simulink library "hal"  (Simulink 8.2)
settings: Solver=ode45  SolverMode=SingleTasking  StartTime=0.0  StopTime=10.0  RelTol=1e-3
PostLoadFcn:
  | , if any(exist('dsrtsu_mdlpostloadfcn', 'file') == [2, 3, 6]), try dsrtsu_mdlpostloadfcn('Execute', bdroot); catch fprintf('Error in PostLoadFcn (dsrtsu_mdlpostloadfcn) for model "%s":\n %s\n', bdroot, lasterr); end, end,
values from neighbouring files (symbols this model uses):
  INVALID_ABS1_TIMEOUT = single(0.03)    [hal_def.m]
  INVALID_ABS2_TIMEOUT = single(0.03)    [hal_def.m]
  INVALID_ABS3_TIMEOUT = single(0.03)    [hal_def.m]
  INVALID_ABS4_TIMEOUT = single(0.03)    [hal_def.m]
  INVALID_AC1_TIMEOUT = single(0.3)    [hal_def.m]
  INVALID_BCM1_TIMEOUT = single(0.6)    [hal_def.m]
  INVALID_BCM2_TIMEOUT = single(0.06)    [hal_def.m]
  INVALID_BOOSTER_VAC = uint32(255)    [hal_def.m]
  INVALID_CUR_VEHDECE = uint32(255)    [hal_def.m]
  INVALID_CURBRAKEDECE_REQ = uint32(255)    [hal_def.m]
  INVALID_CURSTEERANG_REQ = uint32(65535)    [hal_def.m]
  INVALID_CURSTEERTQ_REQ = uint32(255)    [hal_def.m]
  INVALID_ECM1_TIMEOUT = single(0.03)    [hal_def.m]
  INVALID_ECM2_TIMEOUT = single(0.03)    [hal_def.m]
  INVALID_ECM3_TIMEOUT = single(0.03)    [hal_def.m]
  INVALID_ECM9_TIMEOUT = single(0.03)    [hal_def.m]
  INVALID_ENG_TORQUE_FRICTIONAL = uint32(255)    [hal_def.m]
  INVALID_ENG_TORQUE_INDICATED = uint32(255)    [hal_def.m]
  INVALID_ENG_TORQUE_INDICATEDCOR = uint32(255)    [hal_def.m]
  INVALID_ENG_TQ_MAX = uint32(65535)    [hal_def.m]
  INVALID_ENG_TQ_MIN = uint32(65535)    [hal_def.m]
  INVALID_EPAS2_TIMEOUT = single(0.03)    [hal_def.m]
  INVALID_EPAS3_TIMEOUT = single(0.03)    [hal_def.m]
  INVALID_EPB1_TIMEOUT = single(0.12)    [hal_def.m]
  INVALID_EPS_BATTVOLT = uint32(251)    [hal_def.m]
  INVALID_ESC_BATTVOLT = uint32(251)    [hal_def.m]
  INVALID_GRADE = uint32(255)    [hal_def.m]
  INVALID_HCU3_TIMEOUT = single(0.03)    [hal_def.m]
  INVALID_HCU4_TIMEOUT = single(0.03)    [hal_def.m]
  INVALID_HMI1_TIMEOUT = single(0.03)    [hal_def.m]
  INVALID_HMI2_TIMEOUT = single(0.03)    [hal_def.m]
  INVALID_LAT_ACC = uint32(255)    [hal_def.m]
  INVALID_LONG_ACC = uint32(255)    [hal_def.m]
  INVALID_MC_PRESSURE = uint32(2047)    [hal_def.m]
  INVALID_METER1_TIMEOUT = single(0.3)    [hal_def.m]
  INVALID_METER3_TIMEOUT = single(0.3)    [hal_def.m]
  INVALID_METER_VEHSPD = uint32(2048)    [hal_def.m]
  INVALID_ODO_METER = uint32(1000000)    [hal_def.m]
  INVALID_OUTSIDE_TEMP = uint32(96)    [hal_def.m]
  INVALID_PARKBRAKEBIND_STAT = uint32(3)    [hal_def.m]
  INVALID_SAS1_TIMEOUT = single(0.03)    [hal_def.m]
  INVALID_SAS_ANGLE = uint32(65535)    [hal_def.m]
  INVALID_SHIFTER_POSN = uint32(6)    [hal_def.m]
  INVALID_TCM1_TIMEOUT = single(0.03)    [hal_def.m]
  INVALID_TCM2_TIMEOUT = single(0.03)    [hal_def.m]
  INVALID_VCU1_TIMEOUT = single(0.03)    [hal_def.m]
  INVALID_VCU2_TIMEOUT = single(0.03)    [hal_def.m]
  INVALID_VEH_CRASH = uint32(15)    [hal_def.m]
  INVALID_VEH_SPD = uint32(2048)    [hal_def.m]
  INVALID_WHEEL_SPD = uint32(16377)    [hal_def.m]
  INVALID_YAW_RATE = uint32(2001)    [hal_def.m]
undefined symbols (not defined in the file or in its folder): C_TASK_5MS_S, FALSE, INVALID_CURPTTORQ_REQ, KHAL_MssgIdObj1_num, KHAL_MssgIdObj2_num, KHAL_MssgIdObjStatus_num, TRUE
libraries: simulink x92
(part 5 of 8)

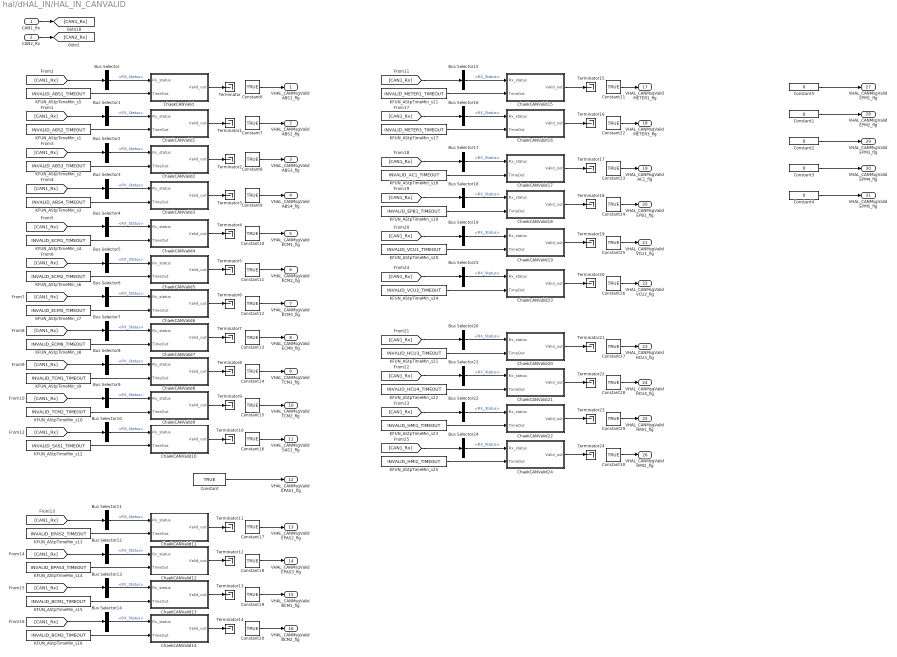
== system hal/dHAL_IN/HAL_IN_CANVALID ==
  CAN1_Rx : Inport
  CAN2_Rx : Inport  Port=2
  Bus Selector : BusSelector  OutputSignals=ABS1.RX_Status
  Bus Selector1 : BusSelector  OutputSignals=ABS2.RX_Status
  Bus Selector10 : BusSelector  OutputSignals=SAS1.RX_Status
  Bus Selector11 : BusSelector  OutputSignals=EPAS2.RX_Status
  Bus Selector12 : BusSelector  OutputSignals=EPAS3.RX_Status
  Bus Selector13 : BusSelector  OutputSignals=BCM1.RX_Status
  Bus Selector14 : BusSelector  OutputSignals=BCM2.RX_Status
  Bus Selector15 : BusSelector  OutputSignals=Meter1.RX_Status
  Bus Selector16 : BusSelector  OutputSignals=Meter3.RX_Status
  Bus Selector17 : BusSelector  OutputSignals=AC1.RX_Status
  Bus Selector18 : BusSelector  OutputSignals=EPB1.RX_Status
  Bus Selector19 : BusSelector  OutputSignals=VCU1.RX_Status
  Bus Selector2 : BusSelector  OutputSignals=ABS3.RX_Status
  Bus Selector20 : BusSelector  OutputSignals=HCU3.RX_Status
  Bus Selector21 : BusSelector  OutputSignals=HCU4.RX_Status
  Bus Selector22 : BusSelector  OutputSignals=HMI1.RX_Status
  Bus Selector23 : BusSelector  OutputSignals=VCU2.RX_Status
  Bus Selector24 : BusSelector  OutputSignals=HMI2.RX_Status
  Bus Selector3 : BusSelector  OutputSignals=ABS4.RX_Status
  Bus Selector4 : BusSelector  OutputSignals=ECM1.RX_Status
  Bus Selector5 : BusSelector  OutputSignals=ECM2.RX_Status
  Bus Selector6 : BusSelector  OutputSignals=ECM3.RX_Status
  Bus Selector7 : BusSelector  OutputSignals=ECM9.RX_Status
  Bus Selector8 : BusSelector  OutputSignals=TCM1.RX_Status
  Bus Selector9 : BusSelector  OutputSignals=TCM2.RX_Status
  ChaekCANValid : Subsystem
  ChaekCANValid1 : Subsystem
  ChaekCANValid10 : Subsystem
  ChaekCANValid11 : Subsystem
  ChaekCANValid12 : Subsystem
  ChaekCANValid13 : Subsystem
  ChaekCANValid14 : Subsystem
  ChaekCANValid15 : Subsystem
  ChaekCANValid16 : Subsystem
  ChaekCANValid17 : Subsystem
  ChaekCANValid18 : Subsystem
  ChaekCANValid19 : Subsystem
  ChaekCANValid2 : Subsystem
  ChaekCANValid20 : Subsystem
  ChaekCANValid21 : Subsystem
  ChaekCANValid22 : Subsystem
  ChaekCANValid23 : Subsystem
  ChaekCANValid24 : Subsystem
  ChaekCANValid3 : Subsystem
  ChaekCANValid4 : Subsystem
  ChaekCANValid5 : Subsystem
  ChaekCANValid6 : Subsystem
  ChaekCANValid7 : Subsystem
  ChaekCANValid8 : Subsystem
  ChaekCANValid9 : Subsystem
  Constant{,6..30} (26 alike) : Constant  Value=TRUE
  Constant{1..5} (5 alike) : Constant  Value=0
  KFUN_AStpTimeMin_s1 : Constant  Value=INVALID_ABS2_TIMEOUT
  KFUN_AStpTimeMin_s10 : Constant  Value=INVALID_TCM2_TIMEOUT
  KFUN_AStpTimeMin_s11 : Constant  Value=INVALID_METER1_TIMEOUT
  KFUN_AStpTimeMin_s12 : Constant  Value=INVALID_SAS1_TIMEOUT
  KFUN_AStpTimeMin_s13 : Constant  Value=INVALID_EPAS2_TIMEOUT
  KFUN_AStpTimeMin_s14 : Constant  Value=INVALID_EPAS3_TIMEOUT
  KFUN_AStpTimeMin_s15 : Constant  Value=INVALID_BCM1_TIMEOUT
  KFUN_AStpTimeMin_s16 : Constant  Value=INVALID_BCM2_TIMEOUT
  KFUN_AStpTimeMin_s17 : Constant  Value=INVALID_METER3_TIMEOUT
  KFUN_AStpTimeMin_s18 : Constant  Value=INVALID_AC1_TIMEOUT
  KFUN_AStpTimeMin_s19 : Constant  Value=INVALID_EPB1_TIMEOUT
  KFUN_AStpTimeMin_s2 : Constant  Value=INVALID_ABS3_TIMEOUT
  KFUN_AStpTimeMin_s20 : Constant  Value=INVALID_VCU1_TIMEOUT
  KFUN_AStpTimeMin_s21 : Constant  Value=INVALID_HCU3_TIMEOUT
  KFUN_AStpTimeMin_s22 : Constant  Value=INVALID_HCU4_TIMEOUT
  KFUN_AStpTimeMin_s23 : Constant  Value=INVALID_HMI1_TIMEOUT  VectorParams1D=off
  KFUN_AStpTimeMin_s24 : Constant  Value=INVALID_VCU2_TIMEOUT
  KFUN_AStpTimeMin_s25 : Constant  Value=INVALID_HMI2_TIMEOUT  VectorParams1D=off
  KFUN_AStpTimeMin_s3 : Constant  Value=INVALID_ABS4_TIMEOUT
  KFUN_AStpTimeMin_s4 : Constant  Value=INVALID_ECM1_TIMEOUT
  KFUN_AStpTimeMin_s5 : Constant  Value=INVALID_ABS1_TIMEOUT
  KFUN_AStpTimeMin_s6 : Constant  Value=INVALID_ECM2_TIMEOUT
  KFUN_AStpTimeMin_s7 : Constant  Value=INVALID_ECM3_TIMEOUT
  KFUN_AStpTimeMin_s8 : Constant  Value=INVALID_ECM9_TIMEOUT
  KFUN_AStpTimeMin_s9 : Constant  Value=INVALID_TCM1_TIMEOUT
  Terminator{,1..24} (25 alike) : Terminator
  VHAL_CANMsgValidABS1_flg : Outport
  VHAL_CANMsgValidABS2_flg : Outport  Port=2
  VHAL_CANMsgValidABS3_flg : Outport  Port=3
  VHAL_CANMsgValidABS4_flg : Outport  Port=4
  VHAL_CANMsgValidECM1_flg : Outport  Port=5
  VHAL_CANMsgValidECM2_flg : Outport  Port=6
  VHAL_CANMsgValidECM3_flg : Outport  Port=7
  VHAL_CANMsgValidECM9_flg : Outport  Port=8
  VHAL_CANMsgValidTCM1_flg : Outport  Port=9
  VHAL_CANMsgValidTCM2_flg : Outport  Port=10
  VHAL_CANMsgValidSAS1_flg : Outport  Port=11
  VHAL_CANMsgValidEPAS1_flg : Outport  Port=12
  VHAL_CANMsgValidEPAS2_flg : Outport  Port=13
  VHAL_CANMsgValidEPAS3_flg : Outport  Port=14
  VHAL_CANMsgValidBCM1_flg : Outport  Port=15
  VHAL_CANMsgValidBCM2_flg : Outport  Port=16
  VHAL_CANMsgValidMETER1_flg : Outport  Port=17
  VHAL_CANMsgValidMETER3_flg : Outport  Port=18
  VHAL_CANMsgValidAC1_flg : Outport  Port=19
  VHAL_CANMsgValidEPB1_flg : Outport  Port=20
  VHAL_CANMsgValidVCU1_flg : Outport  Port=21
  VHAL_CANMsgValidVCU2_flg : Outport  Port=22
  VHAL_CANMsgValidHCU3_flg : Outport  Port=23
  VHAL_CANMsgValidHCU4_flg : Outport  Port=24
  VHAL_CANMsgValidHMI1_flg : Outport  Port=25
  VHAL_CANMsgValidHMI2_flg : Outport  Port=26
  VHAL_CANMsgValidEPM1_flg : Outport  Port=27
  VHAL_CANMsgValidEPM2_flg : Outport  Port=28
  VHAL_CANMsgValidEPM3_flg : Outport  Port=29
  VHAL_CANMsgValidEPM4_flg : Outport  Port=30
  VHAL_CANMsgValidEPM5_flg : Outport  Port=31
  wires:
  Constant/1 -> VHAL_CANMsgValidEPAS1_flg/1
  Constant3/1 -> VHAL_CANMsgValidEPM4_flg/1
  Constant2/1 -> VHAL_CANMsgValidEPM3_flg/1
  Constant1/1 -> VHAL_CANMsgValidEPM2_flg/1
  Constant5/1 -> VHAL_CANMsgValidEPM1_flg/1
  Constant4/1 -> VHAL_CANMsgValidEPM5_flg/1
  [CAN1_Rx] -> Bus Selector/1
  Bus Selector/1 -> ChaekCANValid/1(Rx_status)  "<RX_Status>"
  KFUN_AStpTimeMin_s5/1 -> ChaekCANValid/2(TimeOut)
  CAN1_Rx/1 -> [CAN1_Rx]
  [CAN1_Rx] -> Bus Selector1/1
  Bus Selector1/1 -> ChaekCANValid1/1(Rx_status)  "<RX_Status>"
  KFUN_AStpTimeMin_s1/1 -> ChaekCANValid1/2(TimeOut)
  [CAN1_Rx] -> Bus Selector2/1
  Bus Selector2/1 -> ChaekCANValid2/1(Rx_status)  "<RX_Status>"
  KFUN_AStpTimeMin_s2/1 -> ChaekCANValid2/2(TimeOut)
  [CAN1_Rx] -> Bus Selector3/1
  Bus Selector3/1 -> ChaekCANValid3/1(Rx_status)  "<RX_Status>"
  KFUN_AStpTimeMin_s3/1 -> ChaekCANValid3/2(TimeOut)
  [CAN1_Rx] -> Bus Selector4/1
  Bus Selector4/1 -> ChaekCANValid4/1(Rx_status)  "<RX_Status>"
  KFUN_AStpTimeMin_s4/1 -> ChaekCANValid4/2(TimeOut)
  [CAN1_Rx] -> Bus Selector5/1
  Bus Selector5/1 -> ChaekCANValid5/1(Rx_status)  "<RX_Status>"
  KFUN_AStpTimeMin_s6/1 -> ChaekCANValid5/2(TimeOut)
  [CAN1_Rx] -> Bus Selector6/1
  Bus Selector6/1 -> ChaekCANValid6/1(Rx_status)  "<RX_Status>"
  KFUN_AStpTimeMin_s7/1 -> ChaekCANValid6/2(TimeOut)
  [CAN1_Rx] -> Bus Selector7/1
  Bus Selector7/1 -> ChaekCANValid7/1(Rx_status)  "<RX_Status>"
  KFUN_AStpTimeMin_s8/1 -> ChaekCANValid7/2(TimeOut)
  [CAN1_Rx] -> Bus Selector8/1
  Bus Selector8/1 -> ChaekCANValid8/1(Rx_status)  "<RX_Status>"
  KFUN_AStpTimeMin_s9/1 -> ChaekCANValid8/2(TimeOut)
  [CAN1_Rx] -> Bus Selector9/1
  Bus Selector9/1 -> ChaekCANValid9/1(Rx_status)  "<RX_Status>"
  KFUN_AStpTimeMin_s10/1 -> ChaekCANValid9/2(TimeOut)
  [CAN1_Rx] -> Bus Selector10/1
  Bus Selector10/1 -> ChaekCANValid10/1(Rx_status)  "<RX_Status>"
  KFUN_AStpTimeMin_s12/1 -> ChaekCANValid10/2(TimeOut)
  [CAN1_Rx] -> Bus Selector11/1
  Bus Selector11/1 -> ChaekCANValid11/1(Rx_status)  "<RX_Status>"
  KFUN_AStpTimeMin_s13/1 -> ChaekCANValid11/2(TimeOut)
  [CAN1_Rx] -> Bus Selector12/1
  Bus Selector12/1 -> ChaekCANValid12/1(Rx_status)  "<RX_Status>"
  KFUN_AStpTimeMin_s14/1 -> ChaekCANValid12/2(TimeOut)
  [CAN1_Rx] -> Bus Selector13/1
  Bus Selector13/1 -> ChaekCANValid13/1(Rx_status)  "<RX_Status>"
  KFUN_AStpTimeMin_s15/1 -> ChaekCANValid13/2(TimeOut)
  [CAN1_Rx] -> Bus Selector14/1
  Bus Selector14/1 -> ChaekCANValid14/1(Rx_status)  "<RX_Status>"
  KFUN_AStpTimeMin_s16/1 -> ChaekCANValid14/2(TimeOut)
  [CAN1_Rx] -> Bus Selector15/1
  Bus Selector15/1 -> ChaekCANValid15/1(Rx_status)  "<RX_Status>"
  KFUN_AStpTimeMin_s11/1 -> ChaekCANValid15/2(TimeOut)
  [CAN1_Rx] -> Bus Selector16/1
  Bus Selector16/1 -> ChaekCANValid16/1(Rx_status)  "<RX_Status>"
  KFUN_AStpTimeMin_s17/1 -> ChaekCANValid16/2(TimeOut)
  [CAN1_Rx] -> Bus Selector17/1
  Bus Selector17/1 -> ChaekCANValid17/1(Rx_status)  "<RX_Status>"
  KFUN_AStpTimeMin_s18/1 -> ChaekCANValid17/2(TimeOut)
  [CAN1_Rx] -> Bus Selector18/1
  Bus Selector18/1 -> ChaekCANValid18/1(Rx_status)  "<RX_Status>"
  KFUN_AStpTimeMin_s19/1 -> ChaekCANValid18/2(TimeOut)
  [CAN1_Rx] -> Bus Selector19/1
  Bus Selector19/1 -> ChaekCANValid19/1(Rx_status)  "<RX_Status>"
  KFUN_AStpTimeMin_s20/1 -> ChaekCANValid19/2(TimeOut)
  [CAN1_Rx] -> Bus Selector20/1
  Bus Selector20/1 -> ChaekCANValid20/1(Rx_status)  "<RX_Status>"
  KFUN_AStpTimeMin_s21/1 -> ChaekCANValid20/2(TimeOut)
  [CAN1_Rx] -> Bus Selector21/1
  Bus Selector21/1 -> ChaekCANValid21/1(Rx_status)  "<RX_Status>"
  KFUN_AStpTimeMin_s22/1 -> ChaekCANValid21/2(TimeOut)
  [CAN1_Rx] -> Bus Selector22/1
  Bus Selector22/1 -> ChaekCANValid22/1(Rx_status)  "<RX_Status>"
  KFUN_AStpTimeMin_s23/1 -> ChaekCANValid22/2(TimeOut)
  [CAN1_Rx] -> Bus Selector23/1
  Bus Selector23/1 -> ChaekCANValid23/1(Rx_status)  "<RX_Status>"
  KFUN_AStpTimeMin_s24/1 -> ChaekCANValid23/2(TimeOut)
  CAN2_Rx/1 -> [CAN2_Rx]
  [CAN1_Rx] -> Bus Selector24/1
  Bus Selector24/1 -> ChaekCANValid24/1(Rx_status)  "<RX_Status>"
  KFUN_AStpTimeMin_s25/1 -> ChaekCANValid24/2(TimeOut)
  ChaekCANValid/1(Valid_out) -> Terminator/1
  Constant6/1 -> VHAL_CANMsgValidABS1_flg/1
  ChaekCANValid1/1(Valid_out) -> Terminator1/1
  Constant7/1 -> VHAL_CANMsgValidABS2_flg/1
  Constant8/1 -> VHAL_CANMsgValidABS3_flg/1
  ChaekCANValid2/1(Valid_out) -> Terminator2/1
  Constant9/1 -> VHAL_CANMsgValidABS4_flg/1
  ChaekCANValid3/1(Valid_out) -> Terminator3/1
  Constant10/1 -> VHAL_CANMsgValidECM1_flg/1
  ChaekCANValid4/1(Valid_out) -> Terminator4/1
  Constant11/1 -> VHAL_CANMsgValidECM2_flg/1
  ChaekCANValid5/1(Valid_out) -> Terminator5/1
  ChaekCANValid6/1(Valid_out) -> Terminator6/1
  Constant12/1 -> VHAL_CANMsgValidECM3_flg/1
  Constant13/1 -> VHAL_CANMsgValidECM9_flg/1
  ChaekCANValid7/1(Valid_out) -> Terminator7/1
  Constant14/1 -> VHAL_CANMsgValidTCM1_flg/1
  ChaekCANValid8/1(Valid_out) -> Terminator8/1
  Constant15/1 -> VHAL_CANMsgValidTCM2_flg/1
  ChaekCANValid9/1(Valid_out) -> Terminator9/1
  Constant16/1 -> VHAL_CANMsgValidSAS1_flg/1
  ChaekCANValid10/1(Valid_out) -> Terminator10/1
  Constant17/1 -> VHAL_CANMsgValidEPAS2_flg/1
  ChaekCANValid11/1(Valid_out) -> Terminator11/1
  Constant18/1 -> VHAL_CANMsgValidEPAS3_flg/1
  ChaekCANValid12/1(Valid_out) -> Terminator12/1
  Constant19/1 -> VHAL_CANMsgValidBCM1_flg/1
  ChaekCANValid13/1(Valid_out) -> Terminator13/1
  Constant20/1 -> VHAL_CANMsgValidBCM2_flg/1
  ChaekCANValid14/1(Valid_out) -> Terminator14/1
  Constant21/1 -> VHAL_CANMsgValidMETER1_flg/1
  ChaekCANValid15/1(Valid_out) -> Terminator15/1
  Constant22/1 -> VHAL_CANMsgValidMETER3_flg/1
  ChaekCANValid16/1(Valid_out) -> Terminator16/1
  Constant23/1 -> VHAL_CANMsgValidAC1_flg/1
  ChaekCANValid17/1(Valid_out) -> Terminator17/1
  Constant24/1 -> VHAL_CANMsgValidEPB1_flg/1
  ChaekCANValid18/1(Valid_out) -> Terminator18/1
  Constant25/1 -> VHAL_CANMsgValidVCU1_flg/1
  ChaekCANValid19/1(Valid_out) -> Terminator19/1
  Constant26/1 -> VHAL_CANMsgValidVCU2_flg/1
  ChaekCANValid23/1(Valid_out) -> Terminator20/1
  Constant27/1 -> VHAL_CANMsgValidHCU3_flg/1
  ChaekCANValid20/1(Valid_out) -> Terminator21/1
  Constant28/1 -> VHAL_CANMsgValidHCU4_flg/1
  ChaekCANValid21/1(Valid_out) -> Terminator22/1
  Constant29/1 -> VHAL_CANMsgValidHMI1_flg/1
  ChaekCANValid22/1(Valid_out) -> Terminator23/1
  Constant30/1 -> VHAL_CANMsgValidHMI2_flg/1
  ChaekCANValid24/1(Valid_out) -> Terminator24/1

== system hal/dHAL_IN/HAL_IN_EPB ==
  CAN1_Rx : Inport
  BO__928_EPB1__8_EPB : Subsystem
  KFUN_AStpTimeMin_s3 : Constant  Value=INVALID_PARKBRAKEBIND_STAT
  Relational Operator3 : RelationalOperator  Operator===  OutDataTypeStr=boolean
  VHAL_ParkBrakeBindSta_enum : Outport
  VHAL_ParkBrakeBindStaInvalid_flg : Outport  Port=2
  wires:
  [CAN1_Rx] -> BO__928_EPB1__8_EPB/1(CAN1_Rx)
  CAN1_Rx/1 -> [CAN1_Rx]
  BO__928_EPB1__8_EPB/1(PB_BrakeBinStat) -> VHAL_ParkBrakeBindSta_enum/1, Relational Operator3/1
  Relational Operator3/1 -> VHAL_ParkBrakeBindStaInvalid_flg/1
  KFUN_AStpTimeMin_s3/1 -> Relational Operator3/2

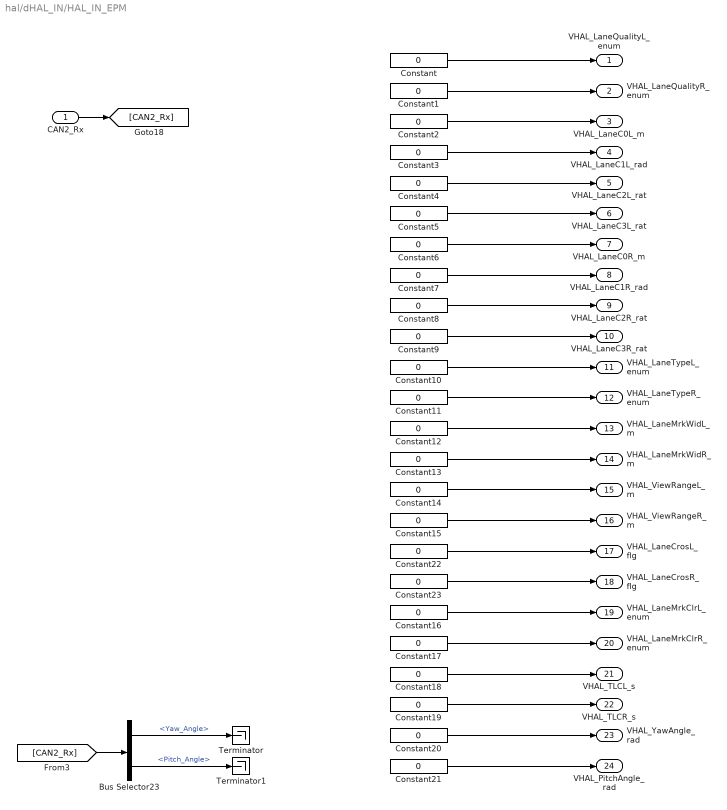
== system hal/dHAL_IN/HAL_IN_EPM ==
  CAN2_Rx : Inport
  Bus Selector23 : BusSelector  OutputSignals=Lane_Details.Yaw_Angle,Lane_Details.Pitch_Angle
  Constant{,1..23} (24 alike) : Constant  Value=0
  Terminator : Terminator
  Terminator1 : Terminator
  VHAL_LaneQualityL_enum : Outport
  VHAL_LaneQualityR_enum : Outport  Port=2
  VHAL_LaneC0L_m : Outport  Port=3
  VHAL_LaneC1L_rad : Outport  Port=4
  VHAL_LaneC2L_rat : Outport  Port=5
  VHAL_LaneC3L_rat : Outport  Port=6
  VHAL_LaneC0R_m : Outport  Port=7
  VHAL_LaneC1R_rad : Outport  Port=8
  VHAL_LaneC2R_rat : Outport  Port=9
  VHAL_LaneC3R_rat : Outport  Port=10
  VHAL_LaneTypeL_enum : Outport  Port=11
  VHAL_LaneTypeR_enum : Outport  Port=12
  VHAL_LaneMrkWidL_m : Outport  Port=13
  VHAL_LaneMrkWidR_m : Outport  Port=14
  VHAL_ViewRangeL_m : Outport  Port=15
  VHAL_ViewRangeR_m : Outport  Port=16
  VHAL_LaneCrosL_flg : Outport  Port=17
  VHAL_LaneCrosR_flg : Outport  Port=18
  VHAL_LaneMrkClrL_enum : Outport  Port=19
  VHAL_LaneMrkClrR_enum : Outport  Port=20
  VHAL_TLCL_s : Outport  Port=21
  VHAL_TLCR_s : Outport  Port=22
  VHAL_YawAngle_rad : Outport  Port=23
  VHAL_PitchAngle_rad : Outport  Port=24
  wires:
  Bus Selector23/2 -> Terminator1/1  "<Pitch_Angle>"
  Bus Selector23/1 -> Terminator/1  "<Yaw_Angle>"
  [CAN2_Rx] -> Bus Selector23/1
  CAN2_Rx/1 -> [CAN2_Rx]
  Constant21/1 -> VHAL_PitchAngle_rad/1
  Constant20/1 -> VHAL_YawAngle_rad/1
  Constant19/1 -> VHAL_TLCR_s/1
  Constant18/1 -> VHAL_TLCL_s/1
  Constant17/1 -> VHAL_LaneMrkClrR_enum/1
  Constant16/1 -> VHAL_LaneMrkClrL_enum/1
  Constant23/1 -> VHAL_LaneCrosR_flg/1
  Constant22/1 -> VHAL_LaneCrosL_flg/1
  Constant15/1 -> VHAL_ViewRangeR_m/1
  Constant14/1 -> VHAL_ViewRangeL_m/1
  Constant13/1 -> VHAL_LaneMrkWidR_m/1
  Constant12/1 -> VHAL_LaneMrkWidL_m/1
  Constant11/1 -> VHAL_LaneTypeR_enum/1
  Constant10/1 -> VHAL_LaneTypeL_enum/1
  Constant9/1 -> VHAL_LaneC3R_rat/1
  Constant8/1 -> VHAL_LaneC2R_rat/1
  Constant7/1 -> VHAL_LaneC1R_rad/1
  Constant6/1 -> VHAL_LaneC0R_m/1
  Constant5/1 -> VHAL_LaneC3L_rat/1
  Constant4/1 -> VHAL_LaneC2L_rat/1
  Constant3/1 -> VHAL_LaneC1L_rad/1
  Constant2/1 -> VHAL_LaneC0L_m/1
  Constant1/1 -> VHAL_LaneQualityR_enum/1
  Constant/1 -> VHAL_LaneQualityL_enum/1

== system hal/dHAL_IN/HAL_IN_HMI ==
  CAN1_Rx : Inport
  BO__1347_HMI1__8_HMI : Subsystem
  Detect Change{,1..2,5..8} (7 alike) : simulink/Logic and Bit Operations/Detect Change  vinit=0  InputProcessing=Inherited  OutDataTypeStr=boolean
  VHAL_AEBEnableH_flg : Outport
  VHAL_FCWEnableH_flg : Outport  Port=2
  VHAL_CSCEnableH_flg : Outport  Port=3
  VHAL_LKAEnableH_flg : Outport  Port=4
  VHAL_MAPAEnableH_flg : Outport  Port=5
  VHAL_LCSEnableH_flg : Outport  Port=6
  VHAL_LFCPilotOnH_flg : Outport  Port=7
  VHAL_LFCPilotCancelH_flg : Outport  Port=8
  VHAL_ACCOnH_flg : Outport  Port=9
  VHAL_ACCCancelH_flg : Outport  Port=10
  VHAL_ACCResSpdIncH_flg : Outport  Port=11
  VHAL_ACCSetSpdDecH_flg : Outport  Port=12
  VHAL_ACCSpdIncH_flg : Outport  Port=13
  VHAL_ACCSpdDecH_flg : Outport  Port=14
  VHAL_ACCTimeGapIncH_flg : Outport  Port=15
  VHAL_ACCTimeGapDecH_flg : Outport  Port=16
  VHAL_IGSAOnH_flg : Outport  Port=17
  VHAL_IGSAResSpdIncH_flg : Outport  Port=18
  VHAL_IGSASetSpdDecH_flg : Outport  Port=19
  VHAL_IGSASwitchModeH_flg : Outport  Port=20
  VHAL_FCWWarningModeH_enum : Outport  Port=21
  VHAL_DefMaxACCSetSpeed_kph : Outport  Port=22
  wires:
  BO__1347_HMI1__8_HMI/22(DefMaxACCSetSpeed) -> VHAL_DefMaxACCSetSpeed_kph/1
  BO__1347_HMI1__8_HMI/21(FCWWarningMode) -> VHAL_FCWWarningModeH_enum/1
  Detect Change8/1 -> VHAL_IGSASetSpdDecH_flg/1
  Detect Change7/1 -> VHAL_IGSAResSpdIncH_flg/1
  Detect Change6/1 -> VHAL_ACCTimeGapIncH_flg/1
  Detect Change5/1 -> VHAL_ACCTimeGapDecH_flg/1
  BO__1347_HMI1__8_HMI/6(ACCSpeedInc) -> VHAL_ACCSpdIncH_flg/1
  BO__1347_HMI1__8_HMI/5(ACCSpeedDec) -> VHAL_ACCSpdDecH_flg/1
  Detect Change2/1 -> VHAL_ACCSetSpdDecH_flg/1
  Detect Change1/1 -> VHAL_ACCResSpdIncH_flg/1
  Detect Change/1 -> VHAL_ACCCancelH_flg/1
  [CAN1_Rx] -> BO__1347_HMI1__8_HMI/1(CAN1_Rx)
  CAN1_Rx/1 -> [CAN1_Rx]
  BO__1347_HMI1__8_HMI/20(MAPAEnable) -> VHAL_MAPAEnableH_flg/1
  BO__1347_HMI1__8_HMI/19(LKAEnable) -> VHAL_LKAEnableH_flg/1
  BO__1347_HMI1__8_HMI/18(LFC_PilotOn) -> VHAL_LFCPilotOnH_flg/1
  BO__1347_HMI1__8_HMI/17(LFC_PilotCancel) -> VHAL_LFCPilotCancelH_flg/1
  BO__1347_HMI1__8_HMI/16(LCSEnable) -> VHAL_LCSEnableH_flg/1
  BO__1347_HMI1__8_HMI/15(IGSASwitchMode) -> VHAL_IGSASwitchModeH_flg/1
  BO__1347_HMI1__8_HMI/14(IGSASet_SpdDec) -> Detect Change8/1
  BO__1347_HMI1__8_HMI/13(IGSARes_SpdInc) -> Detect Change7/1
  BO__1347_HMI1__8_HMI/12(IGSAOn) -> VHAL_IGSAOnH_flg/1
  BO__1347_HMI1__8_HMI/11(FCWEnable) -> VHAL_FCWEnableH_flg/1
  BO__1347_HMI1__8_HMI/10(CSCEnable) -> VHAL_CSCEnableH_flg/1
  BO__1347_HMI1__8_HMI/9(AEBEnable) -> VHAL_AEBEnableH_flg/1
  BO__1347_HMI1__8_HMI/8(ACCTimeGapInc) -> Detect Change6/1
  BO__1347_HMI1__8_HMI/7(ACCTimeGapDec) -> Detect Change5/1
  BO__1347_HMI1__8_HMI/4(ACCSet_SpdDec) -> Detect Change2/1
  BO__1347_HMI1__8_HMI/3(ACCRes_SpdInc) -> Detect Change1/1
  BO__1347_HMI1__8_HMI/2(ACCOn) -> VHAL_ACCOnH_flg/1
  BO__1347_HMI1__8_HMI/1(ACCCancel) -> Detect Change/1

== system hal/dHAL_IN/HAL_IN_RadObjDecoder ==
  CAN2_Rx : Inport
  Bus Selector : BusSelector  OutputSignals=RTICANMMCaptureMessage_1.Status,RTICANMMCaptureMessage_2.Status,RTICANMMCaptureMessage_3.Status,RTICANMMCaptureMessage_4.Status,RTICANMMCaptureMessage_5.Status,RTICANMMCaptureMessage_6.Status,RTICANMMCaptureMessage_7.Status,RTICANMMCaptureMessage_8.Status,RTICANMMCaptureMessage_9.Status,RTICANMMCaptureMessage_10.Status,RTICANMMCaptureMessage_11.Status,RTICANMMCaptureMessage_12.Status,RTICANMMCaptureMessage_13.Status,RTICANMMCaptureMessage_14.Status,RTICANMMCaptureMessage_15.Status,RTICANMMCaptureMessage_16.Status,RTICANMMCaptureMessage_17.Status,RTICANMMCaptureMessage_18.Status,RTICANMMCaptureMessage_19.Status,RTICANMMCaptureMessage_20.Status,RTICANMMCaptureMessage_21.Status,RTICANMMCaptureMessage_22.Status,RTICANMMCaptureMessage_23.Status,RTICANMMCaptureMessage_24.Status,RTICANMMCaptureMessage_25.Status
  Bus Selector1 : BusSelector  OutputSignals=RTICANMMCaptureMessage_1,RTICANMMCaptureMessage_2,RTICANMMCaptureMessage_3,RTICANMMCaptureMessage_4,RTICANMMCaptureMessage_5,RTICANMMCaptureMessage_6,RTICANMMCaptureMessage_7,RTICANMMCaptureMessage_8,RTICANMMCaptureMessage_9,RTICANMMCaptureMessage_10,RTICANMMCaptureMessage_11,RTICANMMCaptureMessage_12,RTICANMMCaptureMessage_13,RTICANMMCaptureMessage_14,RTICANMMCaptureMessage_15,RTICANMMCaptureMessage_16,RTICANMMCaptureMessage_17,RTICANMMCaptureMessage_18,RTICANMMCaptureMessage_19,RTICANMMCaptureMessage_20,RTICANMMCaptureMessage_21,RTICANMMCaptureMessage_22,RTICANMMCaptureMessage_23,RTICANMMCaptureMessage_24,RTICANMMCaptureMessage_25
  Bus Selector2 : BusSelector  OutputSignals=StatusFrame,Frames1,Frames2
  Ground : Ground
  N_of_CANData : Sum  Inputs=+++++++++++++++++++++++++
  RObj_Parser : Subsystem
  RObjectPackFrame : Subsystem  TreatAsAtomicUnit=on
  VHAL_RadNofObjects_num : Outport
  VHAL_MeasCounter_num : Outport  Port=2
  VHAL_SensorRxInvalid_enum : Outport  Port=3
  VHAL_SensorSupplyVoltage_V : Outport  Port=4
  VHAL_SensorDefective_enum : Outport  Port=5
  VHAL_SensorMisaligned_enum : Outport  Port=6
  VHAL_SensorSwitchedOff_enum : Outport  Port=7
  VHAL_SensorExternalDisturbed_enum : Outport  Port=8
  VHAL_SensorOutputReduced_enum : Outport  Port=9
  VHAL_LatDistToborderLeft_m : Outport  Port=10
  VHAL_LatDistToborderRight_m : Outport  Port=11
  VHAL_RadObjRolCountVect40_num : Outport  Port=12
  VHAL_RadObjIDVect40_num : Outport  Port=13
  VHAL_RadObjXDisplVect40_m : Outport  Port=14
  VHAL_RadObjVrelXVect40_mps : Outport  Port=15
  VHAL_RadObjAccelXVect40_mps2 : Outport  Port=16
  VHAL_RadObjYDisplVect40_m : Outport  Port=17
  VHAL_RadObjDynPropVect40_enum : Outport  Port=18
  VHAL_RadObjPExistVect40_enum : Outport  Port=19
  VHAL_RadObjMeasStatVect40_enum : Outport  Port=20
  VHAL_RadObjWidthVect40_m : Outport  Port=21
  VHAL_RadObjLengthVect40_m : Outport  Port=22
  VHAL_RadObjRCSVect40_num : Outport  Port=23
  VHAL_RadObjVrelYVect40_mps : Outport  Port=24
  VHAL_RadObjProbVect40_num : Outport  Port=25
  VHAL_RadWarningLevel_enum : Outport  Port=26
  VHAL_RadWarningObjID_num : Outport  Port=27
  wires:
  RObj_Parser/27(VHAL_RadWarningObjID_num) -> VHAL_RadWarningObjID_num/1
  RObj_Parser/26(VHAL_RadWarningLevel_enum) -> VHAL_RadWarningLevel_enum/1
  RObj_Parser/25(VHAL_RadObjProbVect40_num) -> VHAL_RadObjProbVect40_num/1
  RObj_Parser/24(VHAL_RadObjVrelYVect40_mps) -> VHAL_RadObjVrelYVect40_mps/1
  RObj_Parser/23(VHAL_RadObjRCSVect40_num) -> VHAL_RadObjRCSVect40_num/1
  RObj_Parser/22(VHAL_RadObjLengthVect40_m) -> VHAL_RadObjLengthVect40_m/1
  RObj_Parser/21(VHAL_RadObjWidthVect40_m) -> VHAL_RadObjWidthVect40_m/1
  RObj_Parser/20(VHAL_RadObjMeasStatVect40_enum) -> VHAL_RadObjMeasStatVect40_enum/1
  RObj_Parser/19(VHAL_RadObjPExistVect40_enum) -> VHAL_RadObjPExistVect40_enum/1
  RObj_Parser/18(VHAL_RadObjDynPropVect40_enum) -> VHAL_RadObjDynPropVect40_enum/1
  RObj_Parser/17(VHAL_RadObjYDisplVect40_m) -> VHAL_RadObjYDisplVect40_m/1
  RObj_Parser/16(VHAL_RadObjAccelXVect40_mps2) -> VHAL_RadObjAccelXVect40_mps2/1
  RObj_Parser/15(VHAL_RadObjVrelXVect40_mps) -> VHAL_RadObjVrelXVect40_mps/1
  RObj_Parser/14(VHAL_RadObjXDisplVect40_m) -> VHAL_RadObjXDisplVect40_m/1
  RObj_Parser/13(VHAL_RadObjIDVect40_num) -> VHAL_RadObjIDVect40_num/1
  RObj_Parser/12(VHAL_RadObjRolCountVect40_num) -> VHAL_RadObjRolCountVect40_num/1
  RObj_Parser/11(VHAL_LatDistToborderRight_m) -> VHAL_LatDistToborderRight_m/1
  RObj_Parser/9(VHAL_SensorOutputReduced_enum) -> VHAL_SensorOutputReduced_enum/1
  RObj_Parser/8(VHAL_SensorExternalDisturbed_enum) -> VHAL_SensorExternalDisturbed_enum/1
  RObj_Parser/2(VHAL_MeasCounter_num) -> VHAL_MeasCounter_num/1
  RObj_Parser/10(VHAL_LatDistToborderLeft_m) -> VHAL_LatDistToborderLeft_m/1
  RObj_Parser/6(VHAL_SensorMisaligned_enum) -> VHAL_SensorMisaligned_enum/1
  RObj_Parser/4(VHAL_SensorSupplyVoltage_V) -> VHAL_SensorSupplyVoltage_V/1
  RObj_Parser/7(VHAL_SensorSwitchedOff_enum) -> VHAL_SensorSwitchedOff_enum/1
  RObj_Parser/3(VHAL_SensorRxInvalid_enum) -> VHAL_SensorRxInvalid_enum/1
  RObj_Parser/1(VHAL_RadNofObjects_num) -> VHAL_RadNofObjects_num/1
  RObj_Parser/5(VHAL_SensorDefective_enum) -> VHAL_SensorDefective_enum/1
  [RObj_Frames2] -> RObj_Parser/3(RObj_Frames2)
  [RObj_Frames1] -> RObj_Parser/2(RObj_Frames1)
  [RObj_Status] -> RObj_Parser/1(RObj_Status)
  CAN2_Rx/1 -> Bus Selector/1, Bus Selector1/1
  Bus Selector2/3 -> [RObj_Frames2]  "<Frames2>"
  Bus Selector2/2 -> [RObj_Frames1]  "<Frames1>"
  Bus Selector2/1 -> [RObj_Status]  "<StatusFrame>"
  RObjectPackFrame/1(R_Objects_out) -> Bus Selector2/1
  Bus Selector1/2 -> RObjectPackFrame/3(CaptureMessage2)  "<RTICANMMCaptureMessage_2>"
  Bus Selector1/1 -> RObjectPackFrame/2(CaptureMessage1)  "<RTICANMMCaptureMessage_1>"
  Bus Selector1/8 -> RObjectPackFrame/9(CaptureMessage8)  "<RTICANMMCaptureMessage_8>"
  Bus Selector1/10 -> RObjectPackFrame/11(CaptureMessage10)  "<RTICANMMCaptureMessage_10>"
  Bus Selector1/11 -> RObjectPackFrame/12(CaptureMessage11)  "<RTICANMMCaptureMessage_11>"
  Bus Selector1/12 -> RObjectPackFrame/13(CaptureMessage12)  "<RTICANMMCaptureMessage_12>"
  Bus Selector1/9 -> RObjectPackFrame/10(CaptureMessage9)  "<RTICANMMCaptureMessage_9>"
  Bus Selector1/13 -> RObjectPackFrame/14(CaptureMessage13)  "<RTICANMMCaptureMessage_13>"
  Bus Selector1/22 -> RObjectPackFrame/23(CaptureMessage22)  "<RTICANMMCaptureMessage_22>"
  Bus Selector1/18 -> RObjectPackFrame/19(CaptureMessage18)  "<RTICANMMCaptureMessage_18>"
  Bus Selector1/17 -> RObjectPackFrame/18(CaptureMessage17)  "<RTICANMMCaptureMessage_17>"
  Bus Selector1/23 -> RObjectPackFrame/24(CaptureMessage23)  "<RTICANMMCaptureMessage_23>"
  Bus Selector1/24 -> RObjectPackFrame/25(CaptureMessage24)  "<RTICANMMCaptureMessage_24>"
  Bus Selector1/21 -> RObjectPackFrame/22(CaptureMessage21)  "<RTICANMMCaptureMessage_21>"
  Bus Selector1/19 -> RObjectPackFrame/20(CaptureMessage19)  "<RTICANMMCaptureMessage_19>"
  Bus Selector1/20 -> RObjectPackFrame/21(CaptureMessage20)  "<RTICANMMCaptureMessage_20>"
  Bus Selector1/16 -> RObjectPackFrame/17(CaptureMessage16)  "<RTICANMMCaptureMessage_16>"
  Bus Selector1/14 -> RObjectPackFrame/15(CaptureMessage14)  "<RTICANMMCaptureMessage_14>"
  Bus Selector1/15 -> RObjectPackFrame/16(CaptureMessage15)  "<RTICANMMCaptureMessage_15>"
  Bus Selector1/25 -> RObjectPackFrame/26(CaptureMessage25)  "<RTICANMMCaptureMessage_25>"
  Bus Selector1/5 -> RObjectPackFrame/6(CaptureMessage5)  "<RTICANMMCaptureMessage_5>"
  Bus Selector1/3 -> RObjectPackFrame/4(CaptureMessage3)  "<RTICANMMCaptureMessage_3>"
  Bus Selector1/6 -> RObjectPackFrame/7(CaptureMessage6)  "<RTICANMMCaptureMessage_6>"
  Bus Selector1/7 -> RObjectPackFrame/8(CaptureMessage7)  "<RTICANMMCaptureMessage_7>"
  Bus Selector1/4 -> RObjectPackFrame/5(CaptureMessage4)  "<RTICANMMCaptureMessage_4>"
  N_of_CANData/1 -> RObjectPackFrame/1(CAN_Frames)
  Bus Selector/25 -> N_of_CANData/25  "<Status>"
  Bus Selector/24 -> N_of_CANData/24  "<Status>"
  Bus Selector/23 -> N_of_CANData/23  "<Status>"
  Bus Selector/22 -> N_of_CANData/22  "<Status>"
  Bus Selector/21 -> N_of_CANData/21  "<Status>"
  Bus Selector/20 -> N_of_CANData/20  "<Status>"
  Bus Selector/19 -> N_of_CANData/19  "<Status>"
  Bus Selector/18 -> N_of_CANData/18  "<Status>"
  Bus Selector/17 -> N_of_CANData/17  "<Status>"
  Bus Selector/16 -> N_of_CANData/16  "<Status>"
  Bus Selector/15 -> N_of_CANData/15  "<Status>"
  Bus Selector/14 -> N_of_CANData/14  "<Status>"
  Bus Selector/13 -> N_of_CANData/13  "<Status>"
  Bus Selector/12 -> N_of_CANData/12  "<Status>"
  Bus Selector/11 -> N_of_CANData/11  "<Status>"
  Bus Selector/10 -> N_of_CANData/10  "<Status>"
  Bus Selector/9 -> N_of_CANData/9  "<Status>"
  Bus Selector/8 -> N_of_CANData/8  "<Status>"
  Bus Selector/7 -> N_of_CANData/7  "<Status>"
  Bus Selector/6 -> N_of_CANData/6  "<Status>"
  Bus Selector/5 -> N_of_CANData/5  "<Status>"
  Bus Selector/4 -> N_of_CANData/4  "<Status>"
  Bus Selector/3 -> N_of_CANData/3  "<Status>"
  Bus Selector/2 -> N_of_CANData/2  "<Status>"
  Bus Selector/1 -> N_of_CANData/1  "<Status>"
  Ground/1 -> RObj_Parser/4(RObj_CollDetWarn)

== system hal/dHAL_IN/HAL_IN_SBG ==
  CAN2_Rx : Inport
  Bus Selector23 : BusSelector  OutputSignals=SBG1.SBG_LONGITUDE,SBG1.SBG_LATITUDE,SBG2.SBG_UNDULATION,SBG2.SBG_ALTITUDE,SBG3.SBG_COURSE_ACC,SBG3.SBG_COURSE
  VHAL_LONGIDUTE_deg : Outport
  VHAL_LATITUDE_deg : Outport  Port=2
  VHAL_UNDULATION_m : Outport  Port=3
  VHAL_ALTITUDE_m : Outport  Port=4
  VHAL_COURSEACC_deg : Outport  Port=5
  VHAL_COURSE_deg : Outport  Port=6
  wires:
  CAN2_Rx/1 -> [CAN2_Rx]
  [CAN2_Rx] -> Bus Selector23/1
  Bus Selector23/1 -> VHAL_LONGIDUTE_deg/1  "<SBG_LONGITUDE>"
  Bus Selector23/2 -> VHAL_LATITUDE_deg/1  "<SBG_LATITUDE>"
  Bus Selector23/3 -> VHAL_UNDULATION_m/1  "<SBG_UNDULATION>"
  Bus Selector23/4 -> VHAL_ALTITUDE_m/1  "<SBG_ALTITUDE>"
  Bus Selector23/5 -> VHAL_COURSEACC_deg/1  "<SBG_COURSE_ACC>"
  Bus Selector23/6 -> VHAL_COURSE_deg/1  "<SBG_COURSE>"

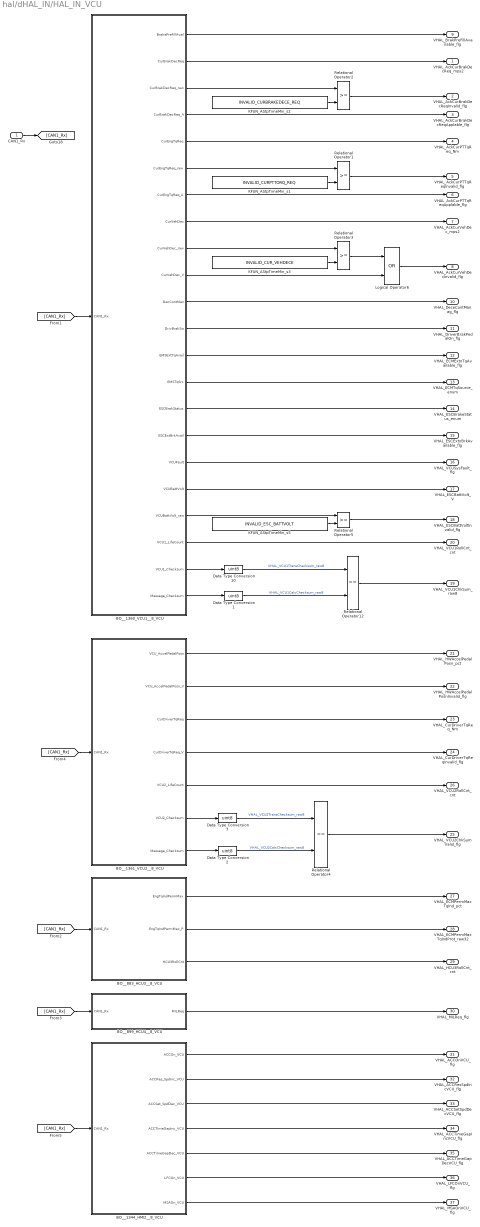
== system hal/dHAL_IN/HAL_IN_VCU ==
  CAN1_Rx : Inport
  BO__1344_HMI2__8_VCU : Subsystem
  BO__1360_VCU1__8_VCU : Subsystem
  BO__1361_VCU2__8_VCU : Subsystem
  BO__883_HCU3__8_VCU : Subsystem
  BO__899_HCU4__8_VCU : Subsystem
  Data Type Conversion{1..3,10} (4 alike) : DataTypeConversion  OutDataTypeStr=uint8
  KFUN_AStpTimeMin_s1 : Constant  Value=INVALID_CURPTTORQ_REQ
  KFUN_AStpTimeMin_s2 : Constant  Value=INVALID_CURBRAKEDECE_REQ
  KFUN_AStpTimeMin_s3 : Constant  Value=INVALID_CUR_VEHDECE
  KFUN_AStpTimeMin_s5 : Constant  Value=INVALID_ESC_BATTVOLT
  Logical Operator6 : Logic  Operator=OR  AllPortsSameDT=off  OutDataTypeStr=boolean
  Relational Operator{1..3,5} (4 alike) : RelationalOperator  OutDataTypeStr=boolean
  Relational Operator12 : RelationalOperator  Operator===  OutDataTypeStr=boolean
  Relational Operator4 : RelationalOperator  Operator===  OutDataTypeStr=boolean
  VHAL_AckCurBrakDecReq_mps2 : Outport
  VHAL_AckCurBrakDecReqInvalid_flg : Outport  Port=2
  VHAL_AckCurBrakDecReqApplable_flg : Outport  Port=3
  VHAL_AckCurPTTqReq_Nm : Outport  Port=4
  VHAL_AckCurPTTqReqInvalid_flg : Outport  Port=5
  VHAL_AckCurPTTqReqApplable_flg : Outport  Port=6
  VHAL_AckCurVehDec_mps2 : Outport  Port=7
  VHAL_AckCurVehDecInvalid_flg : Outport  Port=8
  VHAL_BrakPreFillAvailable_flg : Outport  Port=9
  VHAL_DeceContManag_flg : Outport  Port=10
  VHAL_DriverBrakPedalOn_flg : Outport  Port=11
  VHAL_ECMExtnTqAvailable_flg : Outport  Port=12
  VHAL_ECMTqSource_enum : Outport  Port=13
  VHAL_ESCBrakeStatus_enum : Outport  Port=14
  VHAL_ESCExtnBrkAvailable_flg : Outport  Port=15
  VHAL_VCUSysFault_flg : Outport  Port=16
  VHAL_ESCBattVolt_V : Outport  Port=17
  VHAL_ESCBattVoltInvalid_flg : Outport  Port=18
  VHAL_VCU1ChkSum_raw8 : Outport  Port=19
  VHAL_VCU1RollCnt_cnt : Outport  Port=20
  VHAL_HWAccelPedalPosn_pct : Outport  Port=21
  VHAL_HWAccelPedalPosnInvalid_flg : Outport  Port=22
  VHAL_CurDriverTqReq_Nm : Outport  Port=23
  VHAL_CurDriverTqReqInvalid_flg : Outport  Port=24
  VHAL_VCU2ChkSumValid_flg : Outport  Port=25
  VHAL_VCU2RollCnt_cnt : Outport  Port=26
  VHAL_ECMPermMaxTqInd_pct : Outport  Port=27
  VHAL_ECMPermMaxTqIndProt_raw32 : Outport  Port=28
  VHAL_HCU3RollCnt_cnt : Outport  Port=29
  VHAL_MILReq_flg : Outport  Port=30
  VHAL_ACCOnVCU_flg : Outport  Port=31
  VHAL_ACCResSpdIncVCU_flg : Outport  Port=32
  VHAL_ACCSetSpdDecVCU_flg : Outport  Port=33
  VHAL_ACCTimeGapIncVCU_flg : Outport  Port=34
  VHAL_ACCTimeGapDecVCU_flg : Outport  Port=35
  VHAL_LFCOnVCU_flg : Outport  Port=36
  VHAL_MSAOnVCU_flg : Outport  Port=37
  wires:
  BO__1344_HMI2__8_VCU/7(MSAOn_VCU) -> VHAL_MSAOnVCU_flg/1
  BO__1361_VCU2__8_VCU/4(CurDriverTqReq_V) -> VHAL_CurDriverTqReqInvalid_flg/1
  BO__1361_VCU2__8_VCU/3(CurDriverTqReq) -> VHAL_CurDriverTqReq_Nm/1
  BO__1361_VCU2__8_VCU/5(VCU2_LifeCount) -> VHAL_VCU2RollCnt_cnt/1
  BO__1361_VCU2__8_VCU/2(VCU_AccelPedalPosn_V) -> VHAL_HWAccelPedalPosnInvalid_flg/1
  BO__1361_VCU2__8_VCU/1(VCU_AccelPedalPosn) -> VHAL_HWAccelPedalPosn_pct/1
  BO__1361_VCU2__8_VCU/7(Message_Checksum) -> Data Type Conversion2/1
  BO__1361_VCU2__8_VCU/6(VCU2_Checksum) -> Data Type Conversion3/1
  Data Type Conversion2/1 -> Relational Operator4/2  "VHAL_VCU2CalcChecksum_raw8"
  Data Type Conversion3/1 -> Relational Operator4/1  "VHAL_VCU2TransChecksum_raw8"
  Relational Operator4/1 -> VHAL_VCU2ChkSumValid_flg/1
  [CAN1_Rx] -> BO__1361_VCU2__8_VCU/1(CAN1_Rx)
  BO__1360_VCU1__8_VCU/22(Message_Checksum) -> Data Type Conversion1/1
  BO__1360_VCU1__8_VCU/21(VCU1_Checksum) -> Data Type Conversion10/1
  Data Type Conversion1/1 -> Relational Operator12/2  "VHAL_VCU1CalcChecksum_raw8"
  Data Type Conversion10/1 -> Relational Operator12/1  "VHAL_VCU1TransChecksum_raw8"
  [CAN1_Rx] -> BO__899_HCU4__8_VCU/1(CAN1_Rx)
  [CAN1_Rx] -> BO__883_HCU3__8_VCU/1(CAN1_Rx)
  BO__1360_VCU1__8_VCU/3(CurBrakDecReq_raw) -> Relational Operator2/1
  BO__1360_VCU1__8_VCU/6(CurEngTqReq_raw) -> Relational Operator1/1
  BO__1360_VCU1__8_VCU/9(CurVehDec_raw) -> Relational Operator3/1
  BO__1360_VCU1__8_VCU/19(VCUBattVolt_raw) -> Relational Operator5/1
  [CAN1_Rx] -> BO__1360_VCU1__8_VCU/1(CAN1_Rx)
  CAN1_Rx/1 -> [CAN1_Rx]
  BO__899_HCU4__8_VCU/1(MILReq) -> VHAL_MILReq_flg/1
  BO__883_HCU3__8_VCU/3(HCU3RollCnt) -> VHAL_HCU3RollCnt_cnt/1
  BO__883_HCU3__8_VCU/2(EngTqIndPermMax_P) -> VHAL_ECMPermMaxTqIndProt_raw32/1
  BO__883_HCU3__8_VCU/1(EngTqIndPermMax) -> VHAL_ECMPermMaxTqInd_pct/1
  BO__1360_VCU1__8_VCU/20(VCU1_LifeCount) -> VHAL_VCU1RollCnt_cnt/1
  Relational Operator12/1 -> VHAL_VCU1ChkSum_raw8/1
  KFUN_AStpTimeMin_s5/1 -> Relational Operator5/2
  Relational Operator5/1 -> VHAL_ESCBattVoltInvalid_flg/1
  BO__1360_VCU1__8_VCU/18(VCUBattVolt) -> VHAL_ESCBattVolt_V/1
  BO__1360_VCU1__8_VCU/17(VCUFault) -> VHAL_VCUSysFault_flg/1
  BO__1360_VCU1__8_VCU/16(ESCExtBrkAvail) -> VHAL_ESCExtnBrkAvailable_flg/1
  BO__1360_VCU1__8_VCU/15(ESCBrakStatus) -> VHAL_ESCBrakeStatus_enum/1
  BO__1360_VCU1__8_VCU/14(EMSTqSrc) -> VHAL_ECMTqSource_enum/1
  BO__1360_VCU1__8_VCU/13(EMSExtTqAvail) -> VHAL_ECMExtnTqAvailable_flg/1
  BO__1360_VCU1__8_VCU/12(DrivBrakSw) -> VHAL_DriverBrakPedalOn_flg/1
  BO__1360_VCU1__8_VCU/11(DecContMan) -> VHAL_DeceContManag_flg/1
  BO__1360_VCU1__8_VCU/8(CurVehDec) -> VHAL_AckCurVehDec_mps2/1
  BO__1360_VCU1__8_VCU/5(CurEngTqReq) -> VHAL_AckCurPTTqReq_Nm/1
  BO__1360_VCU1__8_VCU/2(CurBrakDecReq) -> VHAL_AckCurBrakDecReq_mps2/1
  BO__1360_VCU1__8_VCU/10(CurVehDec_V) -> Logical Operator6/2
  KFUN_AStpTimeMin_s3/1 -> Relational Operator3/2
  Relational Operator3/1 -> Logical Operator6/1
  Logical Operator6/1 -> VHAL_AckCurVehDecInvalid_flg/1
  BO__1360_VCU1__8_VCU/7(CurEngTqReq_A) -> VHAL_AckCurPTTqReqApplable_flg/1
  KFUN_AStpTimeMin_s1/1 -> Relational Operator1/2
  Relational Operator1/1 -> VHAL_AckCurPTTqReqInvalid_flg/1
  BO__1360_VCU1__8_VCU/4(CurBrakDecReq_A) -> VHAL_AckCurBrakDecReqApplable_flg/1
  KFUN_AStpTimeMin_s2/1 -> Relational Operator2/2
  Relational Operator2/1 -> VHAL_AckCurBrakDecReqInvalid_flg/1
  BO__1360_VCU1__8_VCU/1(BrakePrefillAvail) -> VHAL_BrakPreFillAvailable_flg/1
  BO__1344_HMI2__8_VCU/1(ACCOn_VCU) -> VHAL_ACCOnVCU_flg/1
  BO__1344_HMI2__8_VCU/2(ACCRes_SpdInc_VCU) -> VHAL_ACCResSpdIncVCU_flg/1
  BO__1344_HMI2__8_VCU/3(ACCSet_SpdDec_VCU) -> VHAL_ACCSetSpdDecVCU_flg/1
  BO__1344_HMI2__8_VCU/5(ACCTimeGapDec_VCU) -> VHAL_ACCTimeGapDecVCU_flg/1
  BO__1344_HMI2__8_VCU/4(ACCTimeGapInc_VCU) -> VHAL_ACCTimeGapIncVCU_flg/1
  BO__1344_HMI2__8_VCU/6(LFCOn_VCU) -> VHAL_LFCOnVCU_flg/1
  [CAN1_Rx] -> BO__1344_HMI2__8_VCU/1(CAN1_Rx)

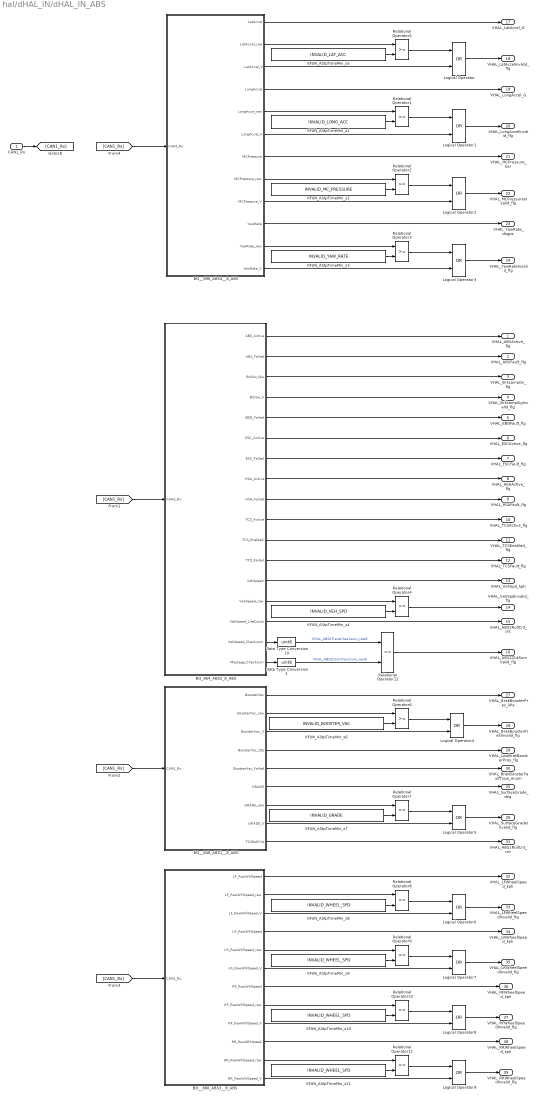
== system hal/dHAL_IN/dHAL_IN_ABS ==
  CAN1_Rx : Inport
  BO_864_ABS2_8_ABS : Subsystem
  BO__848_ABS1__8_ABS : Subsystem
  BO__880_ABS3__8_ABS : Subsystem
  BO__896_ABS4__8_ABS : Subsystem
  Data Type Conversion1 : DataTypeConversion  OutDataTypeStr=uint8
  Data Type Conversion10 : DataTypeConversion  OutDataTypeStr=uint8
  KFUN_AStpTimeMin_s1 : Constant  Value=INVALID_LONG_ACC
  KFUN_AStpTimeMin_s{8..11} (4 alike) : Constant  Value=INVALID_WHEEL_SPD
  KFUN_AStpTimeMin_s2 : Constant  Value=INVALID_MC_PRESSURE
  KFUN_AStpTimeMin_s3 : Constant  Value=INVALID_YAW_RATE
  KFUN_AStpTimeMin_s4 : Constant  Value=INVALID_VEH_SPD
  KFUN_AStpTimeMin_s5 : Constant  Value=INVALID_LAT_ACC
  KFUN_AStpTimeMin_s6 : Constant  Value=INVALID_BOOSTER_VAC
  KFUN_AStpTimeMin_s7 : Constant  Value=INVALID_GRADE
  Logical Operator{,1..9} (10 alike) : Logic  Operator=OR  AllPortsSameDT=off  OutDataTypeStr=boolean
  Relational Operator{1..11} (11 alike) : RelationalOperator  OutDataTypeStr=boolean
  Relational Operator12 : RelationalOperator  Operator===  OutDataTypeStr=boolean
  VHAL_ABSActive_flg : Outport
  VHAL_ABSFault_flg : Outport  Port=2
  VHAL_BrkLampOn_flg : Outport  Port=3
  VHAL_BrkLampSigInvalid_flg : Outport  Port=4
  VHAL_EBDFault_flg : Outport  Port=5
  VHAL_ESCActive_flg : Outport  Port=6
  VHAL_ESCFault_flg : Outport  Port=7
  VHAL_HSAActive_flg : Outport  Port=8
  VHAL_HSAFault_flg : Outport  Port=9
  VHAL_TCSActive_flg : Outport  Port=10
  VHAL_TCSEnabled_flg : Outport  Port=11
  VHAL_TCSFault_flg : Outport  Port=12
  VHAL_VehSpd_kph : Outport  Port=13
  VHAL_VehSpdInvalid_flg : Outport  Port=14
  VHAL_ABS2RollCnt_cnt : Outport  Port=15
  VHAL_ABS2ChkSumValid_flg : Outport  Port=16
  VHAL_LatAccel_G : Outport  Port=17
  VHAL_LatAccelInvalid_flg : Outport  Port=18
  VHAL_LongAccel_G : Outport  Port=19
  VHAL_LongAccelInvalid_flg : Outport  Port=20
  VHAL_MCPressure_bar : Outport  Port=21
  VHAL_MCPressureInvalid_flg : Outport  Port=22
  VHAL_YawRate_degps : Outport  Port=23
  VHAL_YawRateInvalid_flg : Outport  Port=24
  VHAL_SurfaceGrade_deg : Outport  Port=25
  VHAL_SurfaceGradeInvalid_flg : Outport  Port=26
  VHAL_BrakBoosterPres_kPa : Outport  Port=27
  VHAL_BrakBoosterPresInvalid_flg : Outport  Port=28
  VHAL_LowBrakBoosterPres_flg : Outport  Port=29
  VHAL_BrakBoosterFaultType_enum : Outport  Port=30
  VHAL_ABS1RollCnt_cnt : Outport  Port=31
  VHAL_LFWheelSpeed_kph : Outport  Port=32
  VHAL_LFWheelSpeedInvalid_flg : Outport  Port=33
  VHAL_LRWheelSpeed_kph : Outport  Port=34
  VHAL_LRWheelSpeedInvalid_flg : Outport  Port=35
  VHAL_RFWheelSpeed_kph : Outport  Port=36
  VHAL_RFWheelSpeedInvalid_flg : Outport  Port=37
  VHAL_RRWheelSpeed_kph : Outport  Port=38
  VHAL_RRWheelSpeedInvalid_flg : Outport  Port=39
  wires:
  BO__880_ABS3__8_ABS/2(LF_RawWhlSpeed_raw) -> Relational Operator8/1
  BO__880_ABS3__8_ABS/5(LR_RawWhlSpeed_raw) -> Relational Operator9/1
  BO__880_ABS3__8_ABS/8(RF_RawWhlSpeed_raw) -> Relational Operator10/1
  BO__880_ABS3__8_ABS/11(RR_RawWhlSpeed_raw) -> Relational Operator11/1
  BO__848_ABS1__8_ABS/7(GRADE_raw) -> Relational Operator7/1
  Relational Operator6/1 -> Logical Operator4/1
  BO__848_ABS1__8_ABS/2(BoosterVac_raw) -> Relational Operator6/1
  BO_864_ABS2_8_ABS/14(VehSpeed_raw) -> Relational Operator4/1
  BO__896_ABS4__8_ABS/5(LongAcce_raw) -> Relational Operator1/1
  BO__896_ABS4__8_ABS/6(LongAccel_V) -> Logical Operator1/2
  BO__896_ABS4__8_ABS/8(MCPressure_raw) -> Relational Operator2/1
  BO__896_ABS4__8_ABS/12(YawRate_V) -> Logical Operator3/2
  BO__896_ABS4__8_ABS/11(YawRate_raw) -> Relational Operator3/1
  BO__896_ABS4__8_ABS/2(LatAccel_raw) -> Relational Operator5/1
  [CAN1_Rx] -> BO__896_ABS4__8_ABS/1(CAN1_Rx)
  [CAN1_Rx] -> BO__880_ABS3__8_ABS/1(CAN1_Rx)
  [CAN1_Rx] -> BO__848_ABS1__8_ABS/1(CAN1_Rx)
  [CAN1_Rx] -> BO_864_ABS2_8_ABS/1(CAN1_Rx)
  CAN1_Rx/1 -> [CAN1_Rx]
  Data Type Conversion1/1 -> Relational Operator12/2  "VHAL_ABS2CalcChecksum_raw8"
  Data Type Conversion10/1 -> Relational Operator12/1  "VHAL_ABS2TransChecksum_raw8"
  Relational Operator12/1 -> VHAL_ABS2ChkSumValid_flg/1
  BO_864_ABS2_8_ABS/17(Message_Checksum) -> Data Type Conversion1/1
  BO_864_ABS2_8_ABS/16(VehSpeed_Checksum) -> Data Type Conversion10/1
  BO_864_ABS2_8_ABS/15(VehSpeed_LifeCount) -> VHAL_ABS2RollCnt_cnt/1
  Logical Operator9/1 -> VHAL_RRWheelSpeedInvalid_flg/1
  Logical Operator8/1 -> VHAL_RFWheelSpeedInvalid_flg/1
  Logical Operator7/1 -> VHAL_LRWheelSpeedInvalid_flg/1
  Logical Operator6/1 -> VHAL_LFWheelSpeedInvalid_flg/1
  Relational Operator11/1 -> Logical Operator9/1
  KFUN_AStpTimeMin_s11/1 -> Relational Operator11/2
  BO__880_ABS3__8_ABS/12(RR_RawWhlSpeed_V) -> Logical Operator9/2
  BO__880_ABS3__8_ABS/10(RR_RawWhlSpeed) -> VHAL_RRWheelSpeed_kph/1
  Relational Operator10/1 -> Logical Operator8/1
  BO__880_ABS3__8_ABS/7(RF_RawWhlSpeed) -> VHAL_RFWheelSpeed_kph/1
  KFUN_AStpTimeMin_s10/1 -> Relational Operator10/2
  BO__880_ABS3__8_ABS/9(RF_RawWhlSpeed_V) -> Logical Operator8/2
  Relational Operator9/1 -> Logical Operator7/1
  BO__880_ABS3__8_ABS/4(LR_RawWhlSpeed) -> VHAL_LRWheelSpeed_kph/1
  KFUN_AStpTimeMin_s9/1 -> Relational Operator9/2
  BO__880_ABS3__8_ABS/6(LR_RawWhlSpeed_V) -> Logical Operator7/2
  Relational Operator8/1 -> Logical Operator6/1
  BO__880_ABS3__8_ABS/1(LF_RawWhlSpeed) -> VHAL_LFWheelSpeed_kph/1
  KFUN_AStpTimeMin_s8/1 -> Relational Operator8/2
  BO__880_ABS3__8_ABS/3(LF_RawWhlSpeed_V) -> Logical Operator6/2
  BO__848_ABS1__8_ABS/5(BoosterVac_Failed) -> VHAL_BrakBoosterFaultType_enum/1
  BO__848_ABS1__8_ABS/4(BoosterVac_Sta) -> VHAL_LowBrakBoosterPres_flg/1
  Logical Operator4/1 -> VHAL_BrakBoosterPresInvalid_flg/1
  BO__848_ABS1__8_ABS/3(BoosterVac_V) -> Logical Operator4/2
  BO__848_ABS1__8_ABS/1(BoosterVac) -> VHAL_BrakBoosterPres_kPa/1
  KFUN_AStpTimeMin_s6/1 -> Relational Operator6/2
  Logical Operator5/1 -> VHAL_SurfaceGradeInvalid_flg/1
  Relational Operator7/1 -> Logical Operator5/1
  KFUN_AStpTimeMin_s7/1 -> Relational Operator7/2
  BO__848_ABS1__8_ABS/6(GRADE) -> VHAL_SurfaceGrade_deg/1
  BO_864_ABS2_8_ABS/9(HSA_Failed) -> VHAL_HSAFault_flg/1
  BO_864_ABS2_8_ABS/8(HSA_Active) -> VHAL_HSAActive_flg/1
  Relational Operator4/1 -> VHAL_VehSpdInvalid_flg/1
  KFUN_AStpTimeMin_s4/1 -> Relational Operator4/2
  Logical Operator3/1 -> VHAL_YawRateInvalid_flg/1
  Relational Operator3/1 -> Logical Operator3/1
  KFUN_AStpTimeMin_s3/1 -> Relational Operator3/2
  BO__896_ABS4__8_ABS/10(YawRate) -> VHAL_YawRate_degps/1
  Logical Operator2/1 -> VHAL_MCPressureInvalid_flg/1
  Relational Operator2/1 -> Logical Operator2/1
  KFUN_AStpTimeMin_s2/1 -> Relational Operator2/2
  BO__896_ABS4__8_ABS/7(MCPressure) -> VHAL_MCPressure_bar/1
  Logical Operator1/1 -> VHAL_LongAccelInvalid_flg/1
  Relational Operator1/1 -> Logical Operator1/1
  KFUN_AStpTimeMin_s1/1 -> Relational Operator1/2
  BO__896_ABS4__8_ABS/4(LongAccel) -> VHAL_LongAccel_G/1
  Logical Operator/1 -> VHAL_LatAccelInvalid_flg/1
  Relational Operator5/1 -> Logical Operator/1
  BO__896_ABS4__8_ABS/1(LatAccel) -> VHAL_LatAccel_G/1
  KFUN_AStpTimeMin_s5/1 -> Relational Operator5/2
  BO__848_ABS1__8_ABS/8(GRADE_V) -> Logical Operator5/2
  BO__896_ABS4__8_ABS/9(MCPressure_V) -> Logical Operator2/2
  BO__896_ABS4__8_ABS/3(LatAccel_V) -> Logical Operator/2
  BO__848_ABS1__8_ABS/9(TCSRollCnt) -> VHAL_ABS1RollCnt_cnt/1
  BO_864_ABS2_8_ABS/12(TCS_Failed) -> VHAL_TCSFault_flg/1
  BO_864_ABS2_8_ABS/11(TCS_Enabled) -> VHAL_TCSEnabled_flg/1
  BO_864_ABS2_8_ABS/10(TCS_Active) -> VHAL_TCSActive_flg/1
  BO_864_ABS2_8_ABS/7(ESC_Failed) -> VHAL_ESCFault_flg/1
  BO_864_ABS2_8_ABS/6(ESC_Active) -> VHAL_ESCActive_flg/1
  BO_864_ABS2_8_ABS/5(EBD_Failed) -> VHAL_EBDFault_flg/1
  BO_864_ABS2_8_ABS/4(BrkSw_V) -> VHAL_BrkLampSigInvalid_flg/1
  BO_864_ABS2_8_ABS/3(BrkSw_Sta) -> VHAL_BrkLampOn_flg/1
  BO_864_ABS2_8_ABS/2(ABS_Failed) -> VHAL_ABSFault_flg/1
  BO_864_ABS2_8_ABS/1(ABS_Active) -> VHAL_ABSActive_flg/1
  BO_864_ABS2_8_ABS/13(VehSpeed) -> VHAL_VehSpd_kph/1

== system hal/dHAL_IN/dHAL_IN_AC ==
  CAN1_Rx : Inport
  BO__1120_AC1__8_AC : Subsystem
  KFUN_AStpTimeMin_s1 : Constant  Value=INVALID_OUTSIDE_TEMP
  Relational Operator1 : RelationalOperator  OutDataTypeStr=boolean
  VHAL_OutsideTemp_degC : Outport
  VHAL_OutsideTempInvalid_flg : Outport  Port=2
  wires:
  KFUN_AStpTimeMin_s1/1 -> Relational Operator1/2
  BO__1120_AC1__8_AC/2(Sta_Out_Temp_raw) -> Relational Operator1/1
  [CAN1_Rx] -> BO__1120_AC1__8_AC/1(CAN1_Rx)
  CAN1_Rx/1 -> [CAN1_Rx]
  Relational Operator1/1 -> VHAL_OutsideTempInvalid_flg/1
  BO__1120_AC1__8_AC/1(Sta_Out_Temp) -> VHAL_OutsideTemp_degC/1

== system hal/dHAL_IN/dHAL_IN_BCM ==
  CAN1_Rx : Inport
  BO__1008_BCM2__8_BCM : Subsystem
  BO__1056_BCM1__8_BCM : Subsystem
  Compare To Constant : simulink/Logic and Bit Operations/Compare To Constant  relop===  const=5  OutDataTypeStr=boolean  ZeroCross=off
  Compare To Constant1 : simulink/Logic and Bit Operations/Compare To Constant  relop=~=  const=5  OutDataTypeStr=boolean  ZeroCross=off
  Compare To Constant2 : simulink/Logic and Bit Operations/Compare To Constant  relop=~=  const=0  OutDataTypeStr=boolean  ZeroCross=off
  KFUN_AStpTimeMin_s3 : Constant  Value=INVALID_VEH_CRASH
  Logical Operator : Logic  Operator=OR  Inputs=3  AllPortsSameDT=off  OutDataTypeStr=boolean
  Relational Operator3 : RelationalOperator  Operator===  OutDataTypeStr=boolean
  VHAL_KeySwitchStatus_enum : Outport
  VHAL_TurnSignalSwL_flg : Outport  Port=2
  VHAL_TurnSignalSwR_flg : Outport  Port=3
  VHAL_DriverDoorOpen_flg : Outport  Port=4
  VHAL_PassengerDoorOpen_flg : Outport  Port=5
  VHAL_LRDoorOpen_flg : Outport  Port=6
  VHAL_RRDoorOpen_flg : Outport  Port=7
  VHAL_TailGateOpen_flg : Outport  Port=8
  VHAL_AnyDoorOpen_flg : Outport  Port=9
  VHAL_HazardLightSw_flg : Outport  Port=10
  VHAL_VehCrashed_flg : Outport  Port=11
  VHAL_VehCrashedInvalid_flg : Outport  Port=12
  wires:
  [CAN1_Rx] -> BO__1008_BCM2__8_BCM/1(CAN1_Rx)
  [CAN1_Rx] -> BO__1056_BCM1__8_BCM/1(CAN1_Rx)
  CAN1_Rx/1 -> [CAN1_Rx]
  BO__1056_BCM1__8_BCM/6(BCM_LTurnLp_Sta) -> VHAL_TurnSignalSwL_flg/1
  BO__1056_BCM1__8_BCM/9(BCM_RTurnLp_Sta) -> VHAL_TurnSignalSwR_flg/1
  BO__1056_BCM1__8_BCM/4(BCM_Key_Sta) -> VHAL_KeySwitchStatus_enum/1
  BO__1056_BCM1__8_BCM/2(BCM_DDrSw_Sta) -> VHAL_DriverDoorOpen_flg/1
  BO__1056_BCM1__8_BCM/7(BCM_PDrSw_Sta) -> VHAL_PassengerDoorOpen_flg/1
  BO__1056_BCM1__8_BCM/5(BCM_LRDrSw_Sta) -> VHAL_LRDoorOpen_flg/1
  BO__1056_BCM1__8_BCM/8(BCM_RRDrSw_Sta) -> VHAL_RRDoorOpen_flg/1
  BO__1056_BCM1__8_BCM/10(BCM_TGateSw_Sta) -> VHAL_TailGateOpen_flg/1
  BO__1056_BCM1__8_BCM/1(BCM_AllDrSw_Sta) -> VHAL_AnyDoorOpen_flg/1
  BO__1056_BCM1__8_BCM/3(BCM_Hazard_Sta) -> VHAL_HazardLightSw_flg/1
  BO__1008_BCM2__8_BCM/1(BCM_SRS_Crash_Info) -> Compare To Constant/1, Relational Operator3/1, Compare To Constant1/1, Compare To Constant2/1
  Compare To Constant/1 -> VHAL_VehCrashed_flg/1
  KFUN_AStpTimeMin_s3/1 -> Relational Operator3/2
  Relational Operator3/1 -> Logical Operator/1
  Logical Operator/1 -> VHAL_VehCrashedInvalid_flg/1
  Compare To Constant1/1 -> Logical Operator/2
  Compare To Constant2/1 -> Logical Operator/3
